simulink model "fullbridgemosfets"  (Simulink 7.1)
settings: Solver=ode15s  StartTime=0.0  StopTime=10  RelTol=1e-3
libraries: powerlib x16
settings Model: Creator=VIT2  LastModifiedBy=jagan
settings DebuggingCC: SaveWithParameterizedLinksMsg=none  SignalResolutionControl=TryResolveAllWithWarning  MultiTaskDSMMsg=warning  MultiTaskCondExecSysMsg=none  StrictBusMsg=None
settings RTWCC: IncludeERTFirstTime=on
settings GRTTargetCC: TargetFcnLib=ansi_tfl_tmw.mat

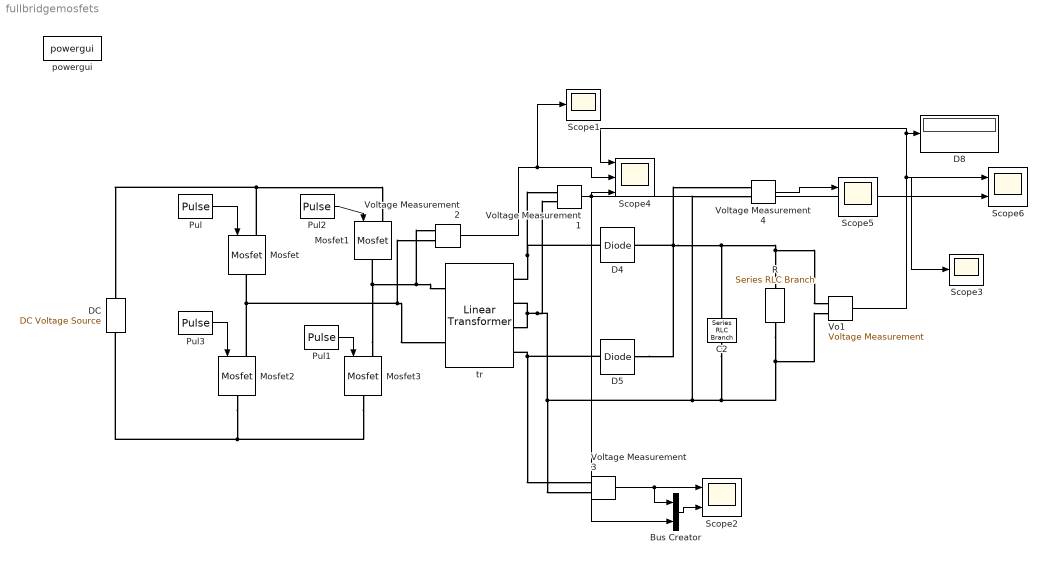
== system fullbridgemosfets ==
  Bus Creator : BusCreator  Inputs=2
  C2 : powerlib/Elements/Series RLC Branch  Orientation=down  DialogController=POWERSYS.PowerSysDialog  PhysicalDomain=powersysdomain  SubClassName=unknown  LeftPortType=p1  RightPortType=p1  LConnTagsString=__new0  RConnTagsString=__new0  BranchType=RLC  Resistance=1  Inductance=1e-3  SetiL0=off  InitialCurrent=0  Capacitance=100e-6  Setx0=off  InitialVoltage=0  Measurements=None
  D4 : powerlib/Power Electronics/Diode  DialogController=POWERSYS.PowerSysDialog  SystemSampleTime=-1  Ron=0.001  Lon=0  Vf=0.8  IC=0  UseSnubber=off  Rs=500  Cs=250e-9  Measurements=off
  D5 : powerlib/Power Electronics/Diode  DialogController=POWERSYS.PowerSysDialog  SystemSampleTime=-1  Ron=0.001  Lon=0  Vf=0.8  IC=0  UseSnubber=off  Rs=500  Cs=250e-9  Measurements=off
  D8 : Display
  DC : powerlib/Electrical Sources/DC Voltage Source  Orientation=up  DialogController=POWERSYS.PowerSysDialog  SystemSampleTime=-1  Amplitude=12  Measurements=None
  Mosfet{,1..3} (4 alike) : powerlib/Power Electronics/Mosfet  Orientation=down  DialogController=POWERSYS.PowerSysDialog  SystemSampleTime=-1  Ron=0.001  Lon=1e-6  Rd=.001  Vfd=0  IC=0  Rs=1e5  Cs=inf  Measurements=off
  Pul : DiscretePulseGenerator  PulseType=Time based  Amplitude=2  Period=20e-3  PulseWidth=50  PhaseDelay=10e-3
  Pul1 : DiscretePulseGenerator  PulseType=Time based  Amplitude=2  Period=20e-3  PulseWidth=50  PhaseDelay=10e-3
  Pul2 : DiscretePulseGenerator  PulseType=Time based  Amplitude=2  Period=20e-3  PulseWidth=50
  Pul3 : DiscretePulseGenerator  PulseType=Time based  Amplitude=2  Period=20e-3  PulseWidth=50
  R : powerlib/Elements/Series RLC Branch  Orientation=down  DialogController=POWERSYS.PowerSysDialog  PhysicalDomain=powersysdomain  SubClassName=unknown  LeftPortType=p1  RightPortType=p1  LConnTagsString=__new0  RConnTagsString=__new0  BranchType=RLC  Resistance=15  Inductance=1e-3  SetiL0=off  InitialCurrent=0  Capacitance=1e-6  Setx0=off  InitialVoltage=0  Measurements=None
  Scope1 : Scope
      settings: TimeRange=0.02  YMin=-2250  YMax=500  MaxDataPoints=5000000
  Scope2 : Scope  NumInputPorts=2
      settings: TimeRange=0.04  YMin=-17.5~-17.5  YMax=17.5~17.5  MaxDataPoints=500000000
  Scope3 : Scope
      settings: TimeRange=0.04  YMax=37.5  SaveName=ScopeData2  MaxDataPoints=5000000
  Scope4 : Scope  NumInputPorts=3
      settings: TimeRange=0.04  YMin=-12.5~-9~-5  YMax=12.5~9~5  SaveName=ScopeData3  MaxDataPoints=500000000
  Scope5 : Scope  NumInputPorts=2
      settings: TimeRange=0.04  YMin=25.41~-15  YMax=25.57~15  SaveName=ScopeData4  MaxDataPoints=500000000
  Scope6 : Scope  NumInputPorts=2
      settings: TimeRange=0.04  YMin=25.41~-15  YMax=25.57~15  SaveName=ScopeData5  MaxDataPoints=500000000
  Vo1 : powerlib/Measurements/Voltage Measurement  DialogController=POWERSYS.PowerSysDialog  SystemSampleTime=-1  PhasorSimulation=off  OutputType=Complex  PSBequivalent=0
  Voltage Measurement{1..4} (4 alike) : powerlib/Measurements/Voltage Measurement  DialogController=POWERSYS.PowerSysDialog  SystemSampleTime=-1  PhasorSimulation=off  OutputType=Complex  PSBequivalent=0
  powergui : powerlib/powergui  SystemSampleTime=-1  SimulationMode=Continuous  SampleTime=50e-6  frequency=60  SPID=off  SwTol=0  Interpol=off  x0status=blocks  echomessages=off  HookPort=off  FunctionMessages=off  EnableUseOfTLC=off  RestoreLinks=warning  frequencyindice=0  Frange=[0:2:500]  Ylog=off  Xlog=on  ShowGrid=off  save=off  variable=ZData  ZoomFFT=on  StartTime=0.0  cycles=1  DisplayStyle=1  fundamental=60  FreqAxis=off  MaxFrequency=1000  frequencyindicesteady=1  RmsSteady=1  display=off  Ts=0  methode=off
  tr : powerlib/Elements/Linear Transformer  DialogController=POWERSYS.PowerSysDialog  PhysicalDomain=powersysdomain  SubClassName=unknown  LeftPortType=p1  RightPortType=p1  LConnTagsString=a|b  RConnTagsString=A|B|C|D  UNITS=pu  NominalPower=[ 10 50]  winding1="[14 0.002  0.0005 ]"  winding2="[10 0.002  0.0002]"  ThreeWindings=on  winding3=[10 0.002 0.0002 ]  RmLm=[ 500 500 ]  Measurements=None  DataType=off
  wires:
  Pul/1 -> Mosfet/1
  Pul1/1 -> Mosfet3/1
  Pul2/1 -> Mosfet1/1
  Pul3/1 -> Mosfet2/1
  Vo1/1 -> Scope3/1, D8/1, Scope4/1, Scope6/1
  Voltage Measurement1/1 -> Bus Creator/2, Scope4/3, Scope6/2
  Voltage Measurement2/1 -> Scope1/1, Scope4/2
  Voltage Measurement3/1 -> Scope2/1, Bus Creator/1
  Voltage Measurement4/1 -> Scope5/1
  Bus Creator/1 -> Scope2/2
  connections:
  Mosfet3/RConn1 -- DC/LConn1 -- Mosfet2/RConn1
  Mosfet3/LConn1 -- tr/LConn1 -- Voltage Measurement2/LConn1 -- Mosfet1/RConn1
  Mosfet2/LConn1 -- tr/LConn2 -- Voltage Measurement2/LConn2 -- Mosfet/RConn1
  Mosfet1/LConn1 -- DC/RConn1 -- Mosfet/LConn1
  D4/LConn1 -- tr/RConn1 -- Voltage Measurement1/LConn1
  C2/RConn1 -- R/RConn1 -- Vo1/LConn2 -- tr/RConn3 -- tr/RConn2 -- Voltage Measurement1/LConn2 -- Voltage Measurement3/LConn2 -- Voltage Measurement4/LConn2
  D5/LConn1 -- tr/RConn4 -- Voltage Measurement3/LConn1
  D4/RConn1 -- R/LConn1 -- Vo1/LConn1 -- C2/LConn1 -- Voltage Measurement4/LConn1 -- D5/RConn1
